simulink model "cascaded_h_bridge_inverter"  (R2023b)
settings: Solver=ode23t  StartTime=0.0  StopTime=0.1  MaxStep=1e-6  RelTol=1e-3
model workspace (MAT data in the model file):
  Vdco = 20
  ma = 0.847307175891
  mf = 104.920699471
libraries: spsIGBTLib x20, simulink x10, spsDCVoltageSourceLib x5, spsCurrentMeasurementLib x1, spsSeriesRLCBranchLib x1, spsTHDLib x1, spsVoltageMeasurementLib x1, sps_lib x1
settings Model: Creator=ixale  LastModifiedBy=ixale
settings DataIOCC: ReturnWorkspaceOutputs=off

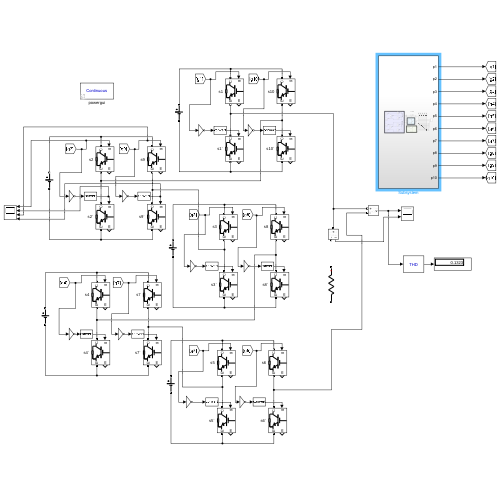
[thumbnail: Simulink's stored preview of the top-level diagram]
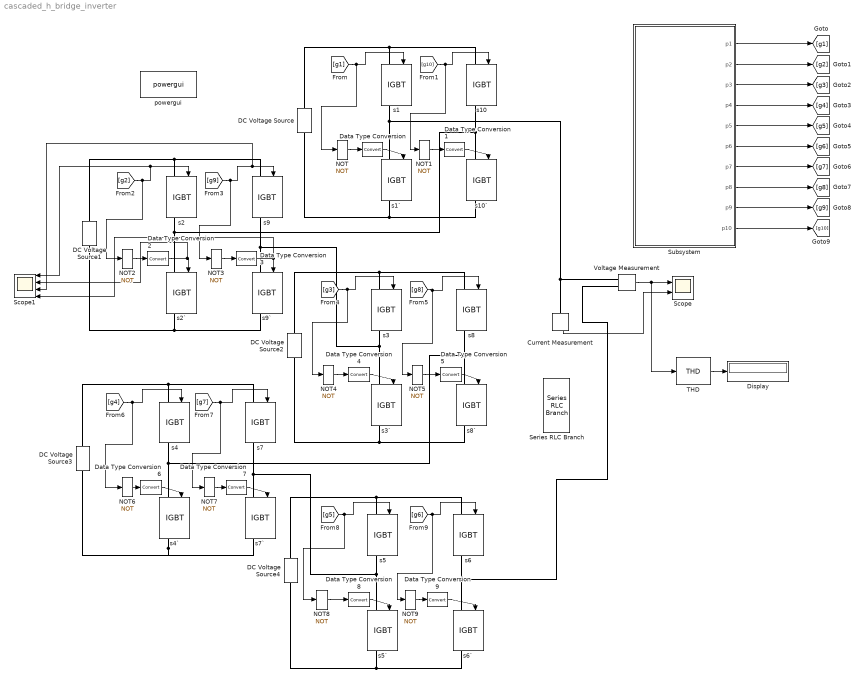
== system cascaded_h_bridge_inverter ==
  Current Measurement : spsCurrentMeasurementLib/Current Measurement  PhasorSimulation=off  OutputType=Complex  PSBequivalent=0
  DC Voltage Source{,1..4} (5 alike) : spsDCVoltageSourceLib/DC Voltage Source  Amplitude=Vdco  Measurements=None
  Data Type Conversion{,1..9} (10 alike) : DataTypeConversion  SaturateOnIntegerOverflow=off  RndMeth=Floor
  Display : Display
  NOT{,1..9} (10 alike) : Logic  Operator=NOT  IconShape=distinctive  AllPortsSameDT=off  OutDataTypeStr=boolean
  Scope : Scope  NumInputPorts=2
  Scope1 : Scope  NumInputPorts=4
  Series RLC Branch : spsSeriesRLCBranchLib/Series RLC Branch  LConnTagsString=__new0  RConnTagsString=__new0  BranchType=R  Resistance=0.1  Inductance=1e-6  SetiL0=off  InitialCurrent=0  Capacitance=1e-6  Setx0=off  InitialVoltage=0  Measurements=None
  Subsystem : Subsystem
  THD : spsTHDLib/THD  Freq=50  Ts=0
  Voltage Measurement : spsVoltageMeasurementLib/Voltage Measurement  PhasorSimulation=off  OutputType=Complex  PSBequivalent=0
  powergui : sps_lib/powergui  Priority=1  SimulationMode=Continuous  SampleTime=1e-6  frequency=60  Iterations=50  frequencyindice=0  Pbase=100e6  ErrMax=1e-4  UnitsV=kV  UnitsW=MW  buscounter=0  FunctionMessages=off  echomessages=off  EnableUseOfTLC=off  CurrentSourceSwitches=off  DisableSnubberDevices=off  DisableRonSwitches=off  DisableVfSwitches=off  DisplayEquations=off  AutomaticDiscreteSolvers=off  SolverType=Tustin/Backward Euler (TBE)  Interpol=off  ExternalGateDelay=off  methode=off  Ts=100  x0status=blocks  SPID=on  SwTol=0  HookPort=off  NonlinearTolerance=1e-4  nMaxIteration=100  ContinueOnMaxIteration=off  RestoreLinks=warning  ResistiveCurrentMeasurement=off  Frange=[0:2:500]  Ylog=off  Xlog=on  ShowGrid=off  save=off  variable=ZData  structure=0  ZoomFFT=off  StartTime=0.0  cycles=1  DisplayStyle=1  fundamental=60  FreqAxis=off  MaxFrequency=1000  frequencyindicesteady=1  RmsSteady=1  display=off
  s{1..10} (10 alike) : spsIGBTLib/IGBT  Ron=0.001  Lon=0  Vf=1  Tf=1e-6  Tt=2e-6  IC=0  Rs=1e5  Cs=inf  Measurements=on
  s10` : spsIGBTLib/IGBT  Ron=0.001  Lon=0  Vf=1  Tf=1e-6  Tt=2e-6  IC=0  Rs=1e5  Cs=inf  Measurements=on
  s1` : spsIGBTLib/IGBT  Ron=0.001  Lon=0  Vf=1  Tf=1e-6  Tt=2e-6  IC=0  Rs=1e5  Cs=inf  Measurements=on
  s2` : spsIGBTLib/IGBT  Ron=0.001  Lon=0  Vf=1  Tf=1e-6  Tt=2e-6  IC=0  Rs=1e5  Cs=inf  Measurements=on
  s3` : spsIGBTLib/IGBT  Ron=0.001  Lon=0  Vf=1  Tf=1e-6  Tt=2e-6  IC=0  Rs=1e5  Cs=inf  Measurements=on
  s4` : spsIGBTLib/IGBT  Ron=0.001  Lon=0  Vf=1  Tf=1e-6  Tt=2e-6  IC=0  Rs=1e5  Cs=inf  Measurements=on
  s5` : spsIGBTLib/IGBT  Ron=0.001  Lon=0  Vf=1  Tf=1e-6  Tt=2e-6  IC=0  Rs=1e5  Cs=inf  Measurements=on
  s6` : spsIGBTLib/IGBT  Ron=0.001  Lon=0  Vf=1  Tf=1e-6  Tt=2e-6  IC=0  Rs=1e5  Cs=inf  Measurements=on
  s7` : spsIGBTLib/IGBT  Ron=0.001  Lon=0  Vf=1  Tf=1e-6  Tt=2e-6  IC=0  Rs=1e5  Cs=inf  Measurements=on
  s8` : spsIGBTLib/IGBT  Ron=0.001  Lon=0  Vf=1  Tf=1e-6  Tt=2e-6  IC=0  Rs=1e5  Cs=inf  Measurements=on
  s9` : spsIGBTLib/IGBT  Ron=0.001  Lon=0  Vf=1  Tf=1e-6  Tt=2e-6  IC=0  Rs=1e5  Cs=inf  Measurements=on
  wires:
  Voltage Measurement/1 -> THD/1, Scope/1
  Subsystem/1(p1) -> [g1]
  Subsystem/2(p2) -> [g2]
  Subsystem/4(p4) -> [g4]
  Subsystem/3(p3) -> [g3]
  Subsystem/5(p5) -> [g5]
  Subsystem/6(p6) -> [g6]
  Subsystem/7(p7) -> [g7]
  Subsystem/8(p8) -> [g8]
  Subsystem/9(p9) -> [g9]
  Subsystem/10(p10) -> [g10]
  [g1] -> NOT/1, s1/1
  NOT/1 -> Data Type Conversion/1
  [g10] -> NOT1/1, s10/1
  NOT1/1 -> Data Type Conversion1/1
  [g2] -> NOT2/1, s2/1, Scope1/1
  [g9] -> NOT3/1, Scope1/3, s9/1
  [g8] -> s8/1, NOT5/1
  [g3] -> s3/1, NOT4/1
  [g4] -> s4/1, NOT6/1
  [g7] -> NOT7/1, s7/1
  [g6] -> s6/1, NOT9/1
  [g5] -> s5/1, NOT8/1
  NOT2/1 -> Data Type Conversion2/1
  NOT3/1 -> Data Type Conversion3/1
  NOT4/1 -> Data Type Conversion4/1
  NOT5/1 -> Data Type Conversion5/1
  NOT6/1 -> Data Type Conversion6/1
  NOT7/1 -> Data Type Conversion7/1
  NOT8/1 -> Data Type Conversion8/1
  NOT9/1 -> Data Type Conversion9/1
  Current Measurement/1 -> Scope/2
  Data Type Conversion/1 -> s1`/1
  Data Type Conversion1/1 -> s10`/1
  Data Type Conversion2/1 -> Scope1/2, s2`/1
  Data Type Conversion3/1 -> Scope1/4, s9`/1
  Data Type Conversion4/1 -> s3`/1
  Data Type Conversion5/1 -> s8`/1
  Data Type Conversion6/1 -> s4`/1
  Data Type Conversion7/1 -> s7`/1
  Data Type Conversion8/1 -> s5`/1
  Data Type Conversion9/1 -> s6`/1
  THD/1 -> Display/1
  connections:
  DC Voltage Source/RConn1 -- s10/LConn1 -- s1/LConn1
  DC Voltage Source/LConn1 -- s10`/RConn1 -- s1`/RConn1
  s1/RConn1 -- Voltage Measurement/LConn1 -- Current Measurement/LConn1 -- s1`/LConn1
  s2/RConn1 -- s10`/LConn1 -- s10/RConn1 -- s2`/LConn1
  s9/LConn1 -- DC Voltage Source1/RConn1 -- s2/LConn1
  s9`/RConn1 -- s2`/RConn1 -- DC Voltage Source1/LConn1
  s8/LConn1 -- DC Voltage Source2/RConn1 -- s3/LConn1
  s8`/RConn1 -- s3`/RConn1 -- DC Voltage Source2/LConn1
  DC Voltage Source3/RConn1 -- s7/LConn1 -- s4/LConn1
  s4`/RConn1 -- s7`/RConn1 -- DC Voltage Source3/LConn1
  s8/RConn1 -- s8`/LConn1 -- s4`/LConn1 -- s4/RConn1
  s9/RConn1 -- s9`/LConn1 -- s3`/LConn1 -- s3/RConn1
  s6/LConn1 -- DC Voltage Source4/RConn1 -- s5/LConn1
  s6`/RConn1 -- s5`/RConn1 -- DC Voltage Source4/LConn1
  s7/RConn1 -- s5`/LConn1 -- s5/RConn1 -- s7`/LConn1
  s6/RConn1 -- Voltage Measurement/LConn2 -- s6`/LConn1

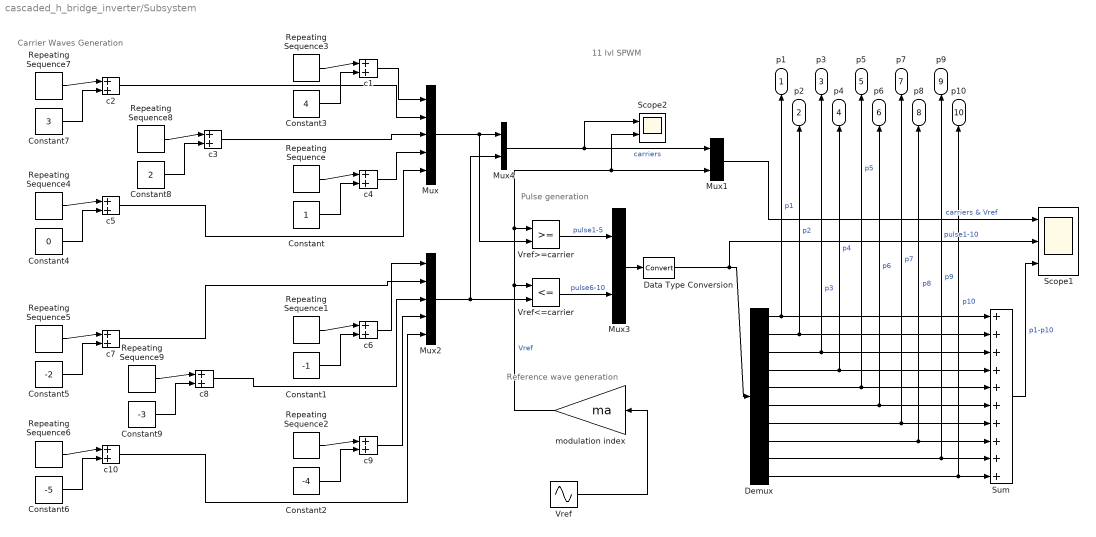
== system cascaded_h_bridge_inverter/Subsystem ==
  note: 11 lvl SPWM
  note: Carrier Waves Generation
  note: Pulse generation
  note: Reference wave generation
  Constant : Constant
  Constant1 : Constant  Value=-1
  Constant2 : Constant  Value=-4
  Constant3 : Constant  Value=4
  Constant4 : Constant  Value=0
  Constant5 : Constant  Value=-2
  Constant6 : Constant  Value=-5
  Constant7 : Constant  Value=3
  Constant8 : Constant  Value=2
  Constant9 : Constant  Value=-3
  Data Type Conversion : DataTypeConversion  SaturateOnIntegerOverflow=off  RndMeth=Floor
  Demux : Demux  Outputs=10
  Mux : Mux  Inputs=5
  Mux1 : Mux  Inputs=2
  Mux2 : Mux  Inputs=5
  Mux3 : Mux  Inputs=2
  Mux4 : Mux  Inputs=2
  Repeating Sequence{,1..9} (10 alike) : simulink/Sources/Repeating Sequence  rep_seq_t=[0 0.5 1] / (50 * mf)  rep_seq_y=[0 1 0]
  Scope1 : Scope  NumInputPorts=3
  Scope2 : Scope  NumInputPorts=2
  Sum : Sum  Inputs=++++++++++
  Vref : Sin  Amplitude=5  Frequency=2*pi*50  SampleTime=0
  Vref<=carrier : RelationalOperator  Operator=<=  OutDataTypeStr=boolean  RndMeth=Simplest  InputSameDT=off
  Vref>=carrier : RelationalOperator  OutDataTypeStr=boolean  RndMeth=Simplest  InputSameDT=off
  c{1..10} (10 alike) : Sum  Inputs=|++
  modulation index : Gain  Gain=ma
  p1 : Outport
  p2 : Outport  Port=2
  p3 : Outport  Port=3
  p4 : Outport  Port=4
  p5 : Outport  Port=5
  p6 : Outport  Port=6
  p7 : Outport  Port=7
  p8 : Outport  Port=8
  p9 : Outport  Port=9
  p10 : Outport  Port=10
  wires:
  Repeating Sequence/1 -> c4/1
  Repeating Sequence2/1 -> c9/1
  c6/1 -> Mux2/1
  Vref/1 -> modulation index/1
  Constant3/1 -> c1/2
  Mux1/1 -> Scope1/1  "carriers & Vref"
  Constant1/1 -> c6/2
  Demux/2 -> Sum/2, p2/1  "p2"
  Demux/4 -> p4/1, Sum/4  "p4"
  Mux4/1 -> Scope2/1, Mux1/1  "carriers"
  Mux/1 -> Vref>=carrier/2, Mux4/1
  Constant2/1 -> c9/2
  Vref>=carrier/1 -> Mux3/1  "pulse1-5"
  Vref<=carrier/1 -> Mux3/2  "pulse6-10"
  Constant/1 -> c4/2
  Data Type Conversion/1 -> Scope1/2, Demux/1  "pulse1-10"
  Repeating Sequence1/1 -> c6/1
  Demux/3 -> p3/1, Sum/3  "p3"
  modulation index/1 -> Scope2/2, Mux1/2, Vref>=carrier/1, Vref<=carrier/1  "Vref"
  Repeating Sequence3/1 -> c1/1
  Sum/1 -> Scope1/3  "p1-p10"
  Mux3/1 -> Data Type Conversion/1
  Demux/1 -> Sum/1, p1/1  "p1"
  Mux2/1 -> Mux4/2, Vref<=carrier/2
  c1/1 -> Mux/1
  Repeating Sequence7/1 -> c2/1
  Repeating Sequence5/1 -> c7/1
  Constant4/1 -> c5/2
  Constant6/1 -> c10/2
  c5/1 -> Mux/5
  Constant5/1 -> c7/2
  Constant7/1 -> c2/2
  c7/1 -> Mux2/2
  Repeating Sequence6/1 -> c10/1
  Repeating Sequence4/1 -> c5/1
  Repeating Sequence8/1 -> c3/1
  c8/1 -> Mux2/3
  Constant9/1 -> c8/2
  c3/1 -> Mux/3
  Constant8/1 -> c3/2
  Repeating Sequence9/1 -> c8/1
  c9/1 -> Mux2/4
  c10/1 -> Mux2/5
  c4/1 -> Mux/4
  c2/1 -> Mux/2
  Demux/5 -> p5/1, Sum/5  "p5"
  Demux/6 -> p6/1, Sum/6  "p6"
  Demux/7 -> p7/1, Sum/7  "p7"
  Demux/8 -> p8/1, Sum/8  "p8"
  Demux/9 -> p9/1, Sum/9  "p9"
  Demux/10 -> p10/1, Sum/10  "p10"
